simulink model "bpsk4"  (Simulink 7.6)
settings: Solver=ode45  StartTime=0.0  StopTime=1000  RelTol=1e-3
libraries: dsp_blocks x5, simulink x1
settings Model: Creator=Joshan  LastModifiedBy=Joshan

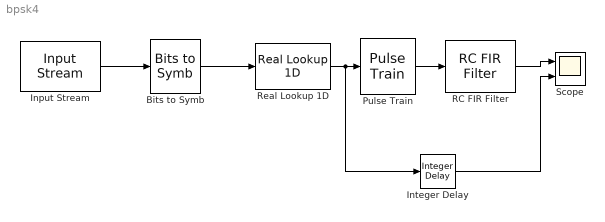
== system bpsk4 ==
  Bits to Symb : dsp_blocks/Conversions/Bits to Symb  SystemSampleTime=-1
  Input Stream : dsp_blocks/Sources//Sinks/Input Stream  SystemSampleTime=-1  period=10  width=1  fname=rand.mat
  Integer Delay : simulink/Discrete/Integer Delay  NumDelays=64  vinit=0.0  samptime=-1
  Pulse Train : dsp_blocks/Conversions/Pulse Train  SystemSampleTime=-1  period=10
  RC FIR Filter : dsp_blocks/Filters/RC FIR Filter  SystemSampleTime=-1  period=10  beta=0.5  root=off  filt_len=128  win_type=on
  Real Lookup 1D : dsp_blocks/Conversions/Real Lookup 1D  SystemSampleTime=-1  table=[-1 1]
  Scope : Scope  NumInputPorts=2
      settings: YMin=-5~-5  YMax=5~5
  wires:
  Bits to Symb/1 -> Real Lookup 1D/1
  Input Stream/1 -> Bits to Symb/1
  Real Lookup 1D/1 -> Pulse Train/1, Integer Delay/1
  Pulse Train/1 -> RC FIR Filter/1
  RC FIR Filter/1 -> Scope/1
  Integer Delay/1 -> Scope/2
